simulink model "OperatingModeAndErrorLogic_RequirementsVerification"  (R2024b)
settings: Solver=FixedStepDiscrete  StartTime=0.0  StopTime=10  FixedStep=ts100ms  RelTol=1e-3
settings Model: Creator=vlenzi  LastModifiedBy=vlenzi
settings RTWCC: GPUComputeCapability=3.5
settings ConfigComp: CovEnable=on  RecordCoverage=on  CovModelRefEnable=on

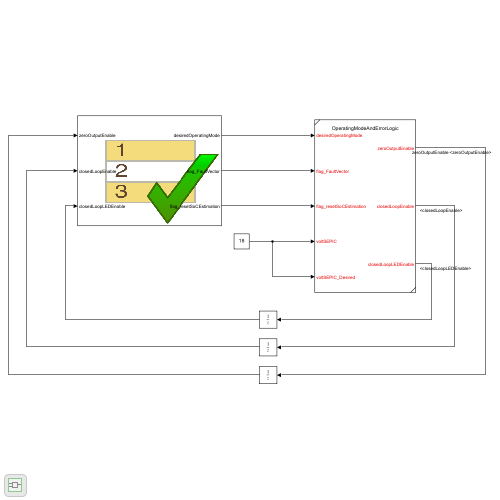
[thumbnail: Simulink's stored preview of the top-level diagram]
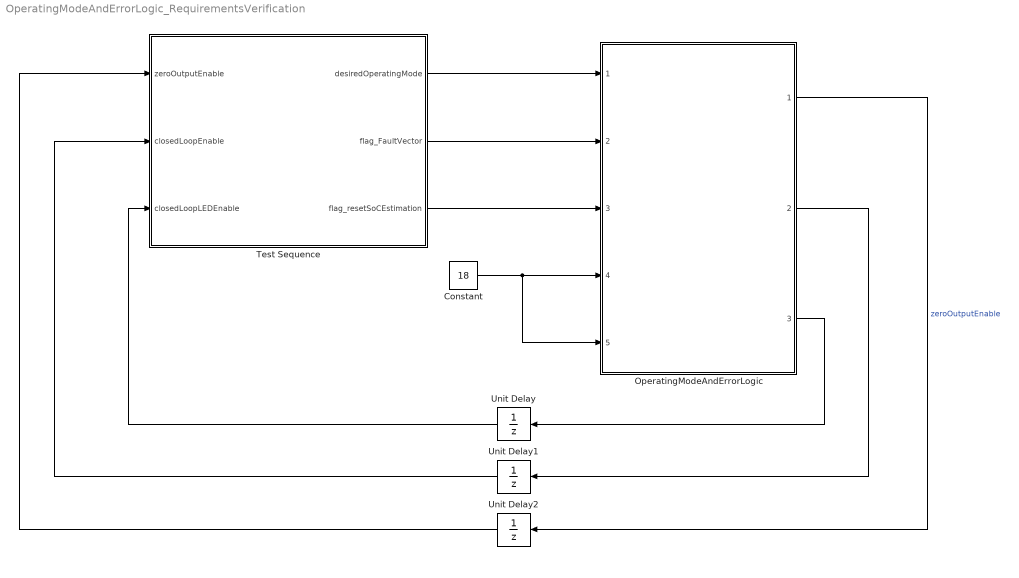
== system OperatingModeAndErrorLogic_RequirementsVerification ==
  Constant : Constant  Value=18
  OperatingModeAndErrorLogic : Subsystem  ReferencedSubsystem=OperatingModeAndErrorLogic
  Test Sequence : Test Sequence  TreatAsAtomicUnit=on
  Unit Delay : UnitDelay  SampleTime=-1  HasFrameUpgradeWarning=on
  Unit Delay1 : UnitDelay  SampleTime=-1  HasFrameUpgradeWarning=on
  Unit Delay2 : UnitDelay  SampleTime=-1  HasFrameUpgradeWarning=on
  wires:
  OperatingModeAndErrorLogic/1 -> Unit Delay2/1  "zeroOutputEnable"
  Constant/1 -> OperatingModeAndErrorLogic/4, OperatingModeAndErrorLogic/5
  OperatingModeAndErrorLogic/2 -> Unit Delay1/1
  Unit Delay/1 -> Test Sequence/3(closedLoopLEDEnable)
  Unit Delay1/1 -> Test Sequence/2(closedLoopEnable)
  Test Sequence/2(flag_FaultVector) -> OperatingModeAndErrorLogic/2
  Test Sequence/1(desiredOperatingMode) -> OperatingModeAndErrorLogic/1
  Test Sequence/3(flag_resetSoCEstimation) -> OperatingModeAndErrorLogic/3
  Unit Delay2/1 -> Test Sequence/1(zeroOutputEnable)
  OperatingModeAndErrorLogic/3 -> Unit Delay/1

== stateflow chart OperatingModeAndErrorLogic_RequirementsVerification/Test Sequence ==
  state step_1
    flag_resetSoCEstimation=true;
    desiredOperatingMode = AllClosedLoop;
    flag_FaultVector =[false false false];
    settings: description=emulating battery estimation behaviour
  state verifyStep1
    verify(zeroOutputEnable ==true)
  state step_2
    flag_resetSoCEstimation=false;
    settings: description=changing operating mode
  state step_2_1
    desiredOperatingMode =AllOpenLoop;
  state verifyStep2_1
    verify((closedLoopEnable && closedLoopLEDEnable) == false )
    verify(zeroOutputEnable==false)
  state step_2_2
    desiredOperatingMode =VoltClosed_CurrOpen;
  state verifyStep2_2
    verify(closedLoopEnable==true &&closedLoopLEDEnable==false)
    verify(zeroOutputEnable==false)
  state step_2_3
    desiredOperatingMode =VoltOpen_CurrClosed;
  state verifyStep2_3
    verify(closedLoopEnable==false &&closedLoopLEDEnable == true)
    verify(zeroOutputEnable==false)
  state step_2_4
    desiredOperatingMode =AllClosedLoop;
  state verifyStep2_4
    verify(closedLoopEnable&&closedLoopLEDEnable == true)
    verify(zeroOutputEnable==false)
  state step_3
    flag_FaultVector =[true true true];
    settings: description=creating fault flag
  state verifyStep3
    verify(zeroOutputEnable==true)
  (default) -> step_1
  step_1 -> verifyStep1 : [
      | after(3,sec)
      | ]
  verifyStep1 -> step_2
  step_2 -> step_2_1
  step_2_1 -> verifyStep2_1 : [
      | after(1,sec)
      | ]
  verifyStep2_1 -> step_2_2
  step_2_2 -> verifyStep2_2 : [
      | after(1,sec)
      | ]
  verifyStep2_2 -> step_2_3
  step_2_3 -> verifyStep2_3 : [
      | after(1,sec)
      | ]
  verifyStep2_3 -> step_2_4
  step_2_4 -> verifyStep2_4 : [
      | after(1,sec)
      | ]
  verifyStep2_4 -> step_3
  step_3 -> verifyStep3 : [
      | after(1,sec)
      | ]
  data: zeroOutputEnable input boolean; closedLoopEnable input boolean; desiredOperatingMode output Enum: operatingMode; flag_FaultVector output boolean; flag_resetSoCEstimation output boolean; closedLoopLEDEnable input boolean
